simulink model "ControleLinear"  (R2019b)
settings: Solver=VariableStepAuto  StartTime=0.0  StopTime=30  RelTol=1e-3
settings Model: Creator=Ploita  LastModifiedBy=Ploita

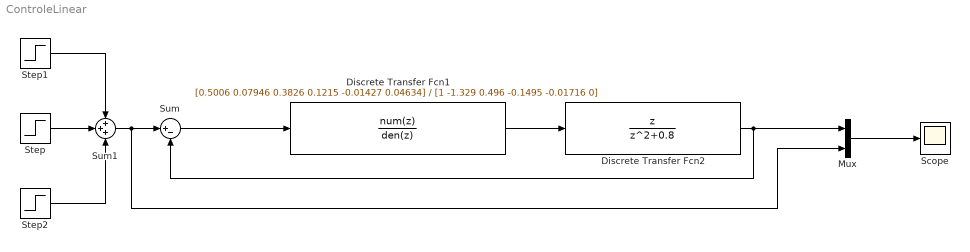
== system ControleLinear ==
  Discrete Transfer Fcn1 : DiscreteTransferFcn  Numerator=[0.5006 0.07946 0.3826 0.1215 -0.01427 0.04634]  Denominator=[1 -1.329 0.496 -0.1495 -0.01716 0]
  Discrete Transfer Fcn2 : DiscreteTransferFcn  Numerator=[ 1 0]  Denominator=[ 1 0 +0.8]
  Mux : Mux  Inputs=2
  Scope : Scope
  Step : Step  Time=8  SampleTime=0
  Step1 : Step  Time=0  After=-2  SampleTime=0
  Step2 : Step  Time=16  After=4  SampleTime=0
  Sum : Sum  Inputs=|+-
  Sum1 : Sum  Inputs=+++
  wires:
  Mux/1 -> Scope/1
  Discrete Transfer Fcn1/1 -> Discrete Transfer Fcn2/1
  Step/1 -> Sum1/2
  Step1/1 -> Sum1/1
  Step2/1 -> Sum1/3
  Sum/1 -> Discrete Transfer Fcn1/1
  Discrete Transfer Fcn2/1 -> Sum/2, Mux/1
  Sum1/1 -> Mux/2, Sum/1
